simulink model "blending_tank_man"  (R2020b)
settings: Solver=FixedStepAuto  StartTime=0.0  StopTime=Inf  RelTol=1e-3
PostLoadFcn:
  | slplc.api.loadDataTypes;
undefined symbols (not defined in the file): BOOL, DINT, slplc
libraries: simulink x1, sldrtlib x1
(part 1 of 4)
CloseFcn:
  | slplc.api.clearDataTypes();
settings Model: Creator=Crystal  LastModifiedBy=Kevin

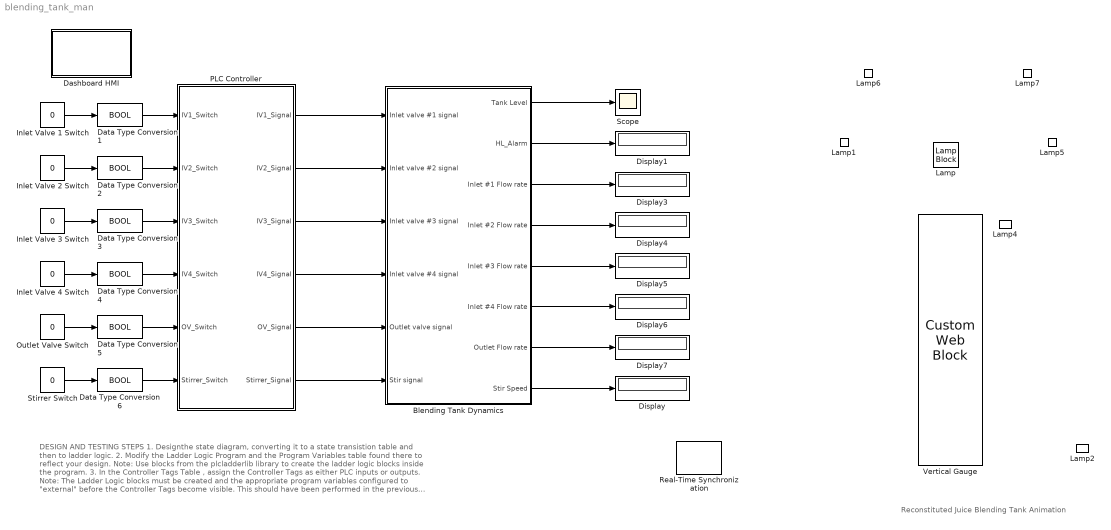
== system blending_tank_man ==
  note: Reconstituted Juice Blending Tank Animation
  note: DESIGN AND TESTING STEPS
      | 1. Designthe state diagram, converting it to a state transistion table and then to ladder logic.
      | 2. Modify the Ladder Logic Program and the Program Variables table found there to reflect your design. Note: Use blocks from the plcladderlib library to create the ladder logic blocks inside the program.
      | 3. In the Controller Tags Table , assign the Controller Tags as either PLC inputs or outputs. Note: The Ladder Logic blocks must be created and the appropriate program variables configured to "external" before the Controller Tags become visible. This should have been performed in the previous step.
      | 4. Wire the physical connections between PLC Controller outputs and the plant inputs. Note: The Controller Tags must be assigned as inputs and outputs before the I/O ports on the PLC controller block can appear. This should have been performed in the previous step.
      | 5. Wire the physical connections between the PLC controller inputs and the (a) plant (b) HMI outputs (optional).
      | 6. Optional: Design the structure of the Dashboard HMI and link the Dashboard components to the HMI outputs and the HMI inputs (from plant).
      | 7. Run the simulation . If HMI is used, control plant behaviour from Dashboard HMI .
  Blending Tank Dynamics : Subsystem
  Dashboard HMI : Subsystem
  Data Type Conversion{1..6} (6 alike) : DataTypeConversion  OutDataTypeStr=BOOL  SaturateOnIntegerOverflow=on  RndMeth=Zero
  Display{,1,3..7} (7 alike) : Display
  Inlet Valve 1 Switch : Constant  Value=0
  Inlet Valve 2 Switch : Constant  Value=0
  Inlet Valve 3 Switch : Constant  Value=0
  Inlet Valve 4 Switch : Constant  Value=0
  Lamp{,1..2,4..7} (7 alike) : LampBlock  LabelPosition=Hide
  Outlet Valve Switch : Constant  Value=0
  PLC Controller : Subsystem  TreatAsAtomicUnit=on  mask{PLCBlockType=PLCController, PLCPOUType=PLC Controller}
      mask init:
      | slplc.callbacks.initController(gcb);
      settings: OpenFcn=slplc.callbacks.openPOUBlock(gcb);
      mask Help: web([docroot '/plccoder/ref/plccontroller' '.html']);
      mask DialogControl PLCBlockTitle Prompt: PLC Controller Block
  Real-Time Synchronization : sldrtlib/Real-Time Synchronization  SampleTime=0.1  MaxMissedTicks=1000  ShowMissedTicks=off  YieldWhenWaiting=off
  Scope : Scope
  Stirrer Switch : Constant  Value=0
  Vertical Gauge : CustomWebBlock  LabelPosition=Hide  ShowInitialText=on  Configuration="{\"components\":[{\"name\":\"LinearScaleComponent\",\"settings\":{\"bounds\":{\"max\":2,\"min\":0,\"tickInterval\":0.1},\"internalTickHeightScaleFactor\":0.5,\"labelColor\":[250,245,199],\"labelFont\":{\"font\":\"Arial\",\"fontSize\":12},\"labelTransparency\":1,\"needleImage\":{\"size\":[21,75],\"src\":\"data:image\\/svg+xml;base64,PHN2ZyB4bWxucz0iaHR0cDovL3d3dy53My5vcmcvMjAwMC9zdmciIHhtbG5zOnhsaW5rPSJodHRwOi8vd3d3LnczLm9yZy8xOTk5L3hsaW5rIiB2aWV3Qm94PSIwIDAgMjEgNzUiPjxkZWZzPjxzdHlsZT4uY2xzLTF7ZmlsbDpub25lO30uY2xzLTJ7aXNvbGF0aW9uOmlzb2xhdGU7fS5jbHMtM3tjbGlwLXBhdGg6dXJsKCNjbGlwLXBhdGgpO30uY2xzLTR7b3BhY2l0eTowLjM7bWl4LWJsZW5kLW1vZGU6bXVsdGlwbHk7fS5jbHMtNXtmaWxsOiNlYjI2Mjk7fTwvc3R5bGU+PGNsaXBQYXRoIGlkPSJjbGlwLXBhdGgiIHRyYW5zZm9y ...(+1928 chars)\",\"srcOrientation\":\"horizontal\"},\"needleOffset\":[-0.01094391244870041,0],\"needleSize\":{\"height\":0.11960078534031414,\"width\":0.7589285714285714},\"position\":[0.015887605042016806,0.06986607142857143,0.8,0.9641544117647058],\"scaleColors\":[],\"scaleColorsSize\":0.2,\"showLabels\":1,\"showMinorTicks\":0,\"showSpanLine\":1,\"showTicks\":1,\"tickColor\":[250,245,200],\"tickTransparency\":1,\"valueBarColor\":[23,89,176],\"valueBarOffset\":0,\"valueBarSize\":0.23,\"valueBarTransparency\":1}},{\"name\":\"BackgroundImageComponent\",\"settings\":{\"image\":{\"size\":[101,380],\"src\":\"data:image\\/svg+xml;base64,PHN2ZyB4bWxucz0iaHR0cDovL3d3dy53My5vcmcvMjAwMC9zdmciIHZpZXdCb3g9IjAgMCAxMDEgMzgwIj48ZGVmcz48c3R5bGU+LmNscy0xe2ZpbGw6IzAwMmI0Mjt9LmNscy0ye2ZpbGw6IzQyNzA4Mjt9LmNscy0ze2ZpbGw6IzdjYTBiMjt9PC9zdHlsZT48L2RlZnM+PHRpdGxlPnZlcnRpY2FsX2dhdWdlX2JhY2tncm91bmRfMTwvdGl0bGU+PGcgaWQ9IkxheWVyXzIiIGRhdGEtbmFtZT0iTGF5ZXIgMiI+PGcgaWQ9IkxheWVyXzEtMiIgZGF0YS1uYW1lPSJMYXllciAxIj48cmVjdCBjbGFzcz0iY2xzLTEiIHg9IjExIiB5PSIxMSIgd2lkdGg9Ijc5IiBoZWlnaHQ9IjM1OCIvPjxwYXRoIGNsYXNzPSJjbHMtMiIgZD0iTTkzLDhIOFYzNzJIOTNaTTExLDM2OVYxMUg5MFYzNjlaIi8+PHBhdGggY2xhc3M9ImNscy0zIiBkPSJNMTAxLDBIMFYzODBIMTAxWk04LDM3MlY4SDkzVjM3MloiLz48L2c+PC9nPjwvc3ZnPg==\",\"srcOrientation\":\"vertical\"},\"position\":[0,0,1,1],\"scaleMode\":\"0\"}},{\"name\":\"ForegroundImageComponent\",\"settings\":{\"image\":{\"size\":[0,0],\"src\":\"default\",\"srcOrientation\":[]},\"isForeground\":1,\"position\":[0,0,1,1],\"scaleMode\":\"0\"}}],\"settings\":{\"BindingType\":\"signal\",\"aspectRatio\":0.26380368098159507,\"fixedAspectRatio\":\"on\",\"orientation\":\"vertical\"},\"type\":\"LinearGauge\"}"
  wires:
  Blending Tank Dynamics/2(HL_Alarm) -> Display1/1
  Blending Tank Dynamics/1(Tank Level) -> Scope/1
  Blending Tank Dynamics/8(Stir Speed) -> Display/1
  Blending Tank Dynamics/3(Inlet #1 Flow rate) -> Display3/1
  Blending Tank Dynamics/4(Inlet #2 Flow rate) -> Display4/1
  Blending Tank Dynamics/5(Inlet #3 Flow rate) -> Display5/1
  Blending Tank Dynamics/6(Inlet #4 Flow rate) -> Display6/1
  Blending Tank Dynamics/7(Outlet Flow rate) -> Display7/1
  PLC Controller/1(IV1_Signal) -> Blending Tank Dynamics/1(Inlet valve #1 signal)
  PLC Controller/2(IV2_Signal) -> Blending Tank Dynamics/2(Inlet valve #2 signal)
  PLC Controller/3(IV3_Signal) -> Blending Tank Dynamics/3(Inlet valve #3 signal)
  PLC Controller/4(IV4_Signal) -> Blending Tank Dynamics/4(Inlet valve #4 signal)
  PLC Controller/6(Stirrer_Signal) -> Blending Tank Dynamics/6(Stir signal)
  PLC Controller/5(OV_Signal) -> Blending Tank Dynamics/5(Outlet valve signal)
  Inlet Valve 1 Switch/1 -> Data Type Conversion1/1
  Data Type Conversion1/1 -> PLC Controller/1(IV1_Switch)
  Data Type Conversion2/1 -> PLC Controller/2(IV2_Switch)
  Inlet Valve 2 Switch/1 -> Data Type Conversion2/1
  Data Type Conversion6/1 -> PLC Controller/6(Stirrer_Switch)
  Stirrer Switch/1 -> Data Type Conversion6/1
  Outlet Valve Switch/1 -> Data Type Conversion5/1
  Data Type Conversion5/1 -> PLC Controller/5(OV_Switch)
  Inlet Valve 4 Switch/1 -> Data Type Conversion4/1
  Data Type Conversion4/1 -> PLC Controller/4(IV4_Switch)
  Inlet Valve 3 Switch/1 -> Data Type Conversion3/1
  Data Type Conversion3/1 -> PLC Controller/3(IV3_Switch)

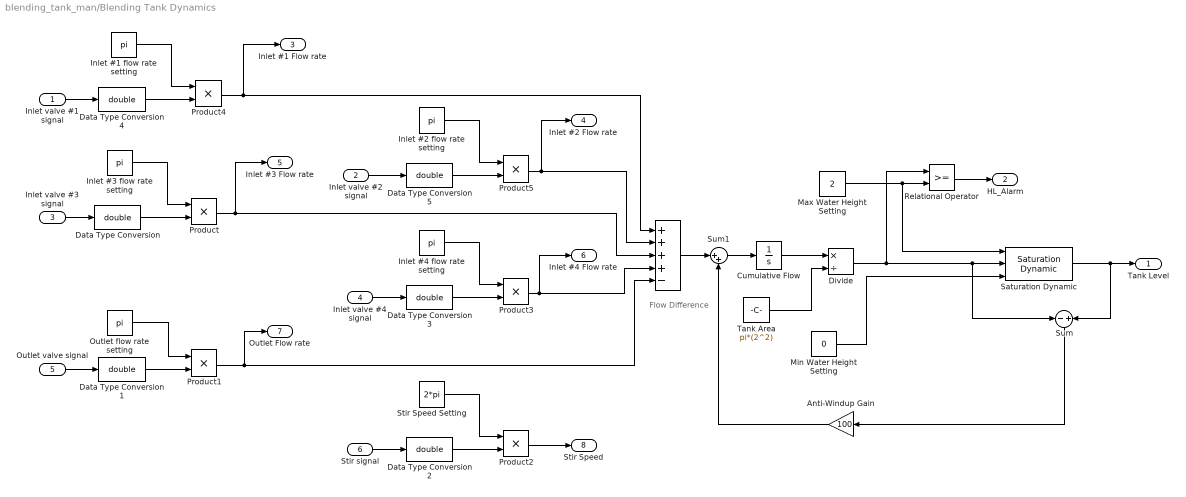
== system blending_tank_man/Blending Tank Dynamics ==
  note: Flow
      | Difference
  Inlet valve #1 signal : Inport
  Inlet valve #2 signal : Inport  Port=2
  Inlet valve #3 signal : Inport  Port=3
  Inlet valve #4 signal : Inport  Port=4
  Outlet valve signal : Inport  Port=5
  Stir signal : Inport  Port=6
  " " : Sum  Inputs=++++-  InputSameDT=on  SaturateOnIntegerOverflow=on  OutDataTypeStr=Inherit: Same as first input
  Anti-Windup Gain : Gain  Gain=100
  Cumulative Flow : Integrator
  Data Type Conversion{,1..5} (6 alike) : DataTypeConversion  OutDataTypeStr=double  SaturateOnIntegerOverflow=on  RndMeth=Zero
  Divide : Product  Inputs=*/
  Inlet #1 flow rate setting : Constant  Value=pi
  Inlet #2 flow rate setting : Constant  Value=pi
  Inlet #3 flow rate setting : Constant  Value=pi
  Inlet #4 flow rate setting : Constant  Value=pi
  Max Water Height Setting : Constant  Value=2
  "Min Water Height Setting " : Constant  Value=0
  Outlet flow rate setting : Constant  Value=pi
  Product{,1..5} (6 alike) : Product
  Relational Operator : RelationalOperator  OutDataTypeStr=boolean  RndMeth=Simplest
  Saturation Dynamic : simulink/Discontinuities/Saturation Dynamic  OutMin=[]  OutMax=[]  OutDataTypeStr=Inherit: Same as second input  OutDataType=fixdt(1, 16)  OutScaling=2^-10  DoSatur=off
  Stir Speed Setting : Constant  Value=2*pi
  Sum : Sum  Inputs=-|+
  Sum1 : Sum  Inputs=|++
  Tank Area : Constant  Value=pi*(2^2)
  Tank Level : Outport  InitialOutput=0  VectorParamsAs1DForOutWhenUnconnected=off
  HL_Alarm : Outport  Port=2
  Inlet #1 Flow rate : Outport  Port=3
  Inlet #2 Flow rate : Outport  Port=4
  Inlet #3 Flow rate : Outport  Port=5
  Inlet #4 Flow rate : Outport  Port=6
  Outlet Flow rate : Outport  Port=7
  Stir Speed : Outport  Port=8
  wires:
  Cumulative Flow/1 -> Divide/1
  Data Type Conversion/1 -> Product/2
  Inlet valve #3 signal/1 -> Data Type Conversion/1
  Outlet valve signal/1 -> Data Type Conversion1/1
  Inlet #3 flow rate setting/1 -> Product/1
  Tank Area/1 -> Divide/2
  Divide/1 -> Sum/1, Saturation Dynamic/2, Relational Operator/1
  Max Water Height Setting/1 -> Relational Operator/2, Saturation Dynamic/1
  "Min Water Height Setting "/1 -> Saturation Dynamic/3
  Relational Operator/1 -> HL_Alarm/1
  Saturation Dynamic/1 -> Sum/2, Tank Level/1
  " "/1 -> Sum1/1
  Sum1/1 -> Cumulative Flow/1
  Sum/1 -> Anti-Windup Gain/1
  Anti-Windup Gain/1 -> Sum1/2
  Stir signal/1 -> Data Type Conversion2/1
  Product2/1 -> Stir Speed/1
  Stir Speed Setting/1 -> Product2/1
  Data Type Conversion2/1 -> Product2/2
  Inlet #4 flow rate setting/1 -> Product3/1
  Inlet valve #4 signal/1 -> Data Type Conversion3/1
  Data Type Conversion3/1 -> Product3/2
  Product5/1 -> " "/2, Inlet #2 Flow rate/1
  Inlet valve #2 signal/1 -> Data Type Conversion5/1
  Inlet #2 flow rate setting/1 -> Product5/1
  Data Type Conversion5/1 -> Product5/2
  Product4/1 -> " "/1, Inlet #1 Flow rate/1
  Inlet #1 flow rate setting/1 -> Product4/1
  Inlet valve #1 signal/1 -> Data Type Conversion4/1
  Data Type Conversion4/1 -> Product4/2
  Product1/1 -> Outlet Flow rate/1, " "/5
  Product3/1 -> " "/4, Inlet #4 Flow rate/1
  Product/1 -> " "/3, Inlet #3 Flow rate/1
  Data Type Conversion1/1 -> Product1/2
  Outlet flow rate setting/1 -> Product1/1

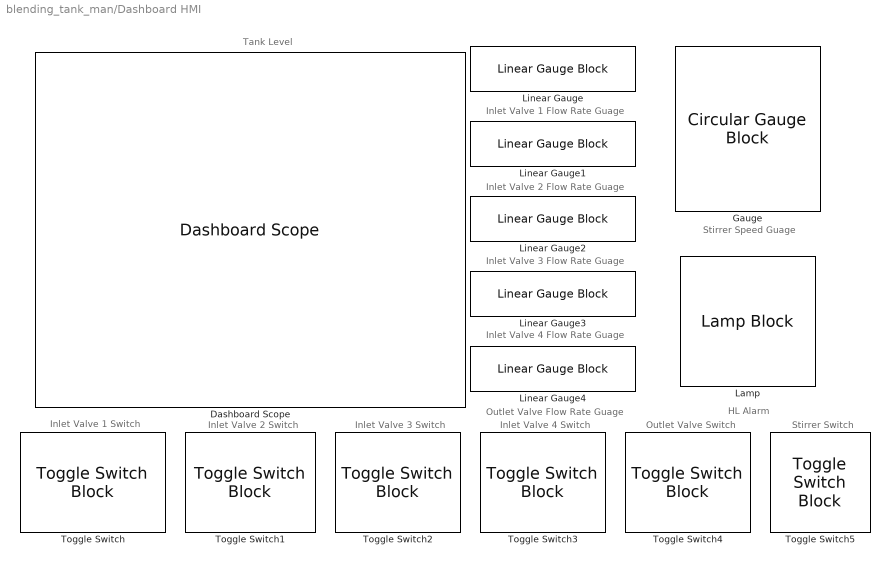
== system blending_tank_man/Dashboard HMI ==
  note: HL Alarm
  note: Stirrer Speed Guage
  note: Tank Level
  note: Inlet Valve 1 Flow Rate Guage
  note: Inlet Valve 2 Flow Rate Guage
  note: Inlet Valve 3 Flow Rate Guage
  note: Inlet Valve 4 Flow Rate Guage
  note: Outlet Valve Flow Rate Guage
  note: Inlet Valve 1 Switch
  note: Inlet Valve 2 Switch
  note: Inlet Valve 3 Switch
  note: Inlet Valve 4 Switch
  note: Outlet Valve Switch
  note: Stirrer Switch
  Dashboard Scope : DashboardScope  TimeSpan=110  Ymin=0  Ymax=2  LegendPosition=Hide  ScaleAtStop=off
  Gauge : CircularGaugeBlock  LabelPosition=Hide  ScaleMax=10  TickInterval=1
  Lamp : LampBlock  LabelPosition=Hide
  Linear Gauge{,1..4} (5 alike) : LinearGaugeBlock  LabelPosition=Hide  ScaleMax=5  TickInterval=0.5
  Toggle Switch{,1..5} (6 alike) : ToggleSwitchBlock  LabelPosition=Hide
      settings: Values={{'Off', 'On'}, [0 1]}

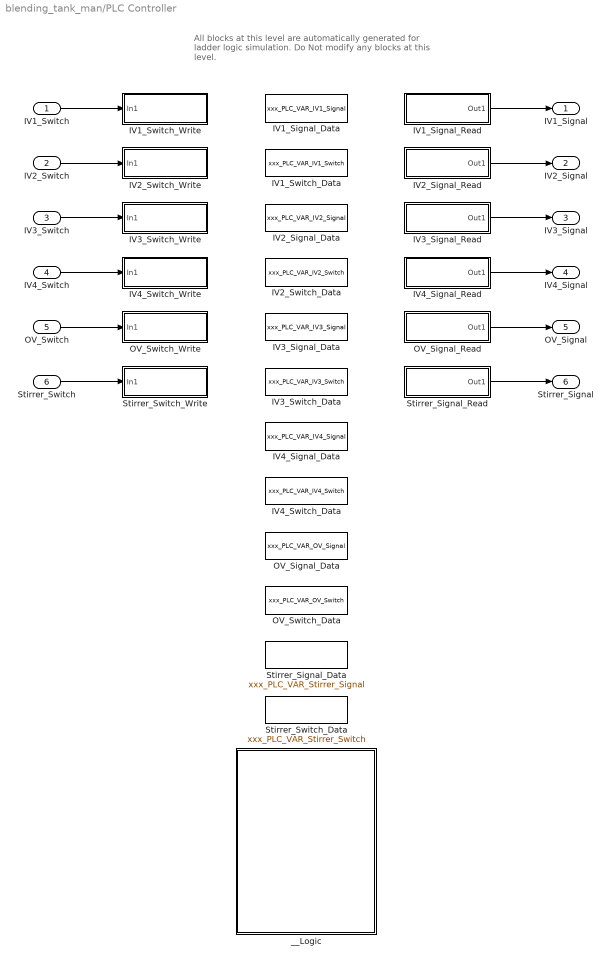
== system blending_tank_man/PLC Controller ==
  note: All blocks at this level are automatically generated for ladder logic simulation.
      | Do Not modify any blocks at this level.
  IV1_Switch : Inport  OutDataTypeStr=BOOL
  IV2_Switch : Inport  Port=2  OutDataTypeStr=BOOL
  IV3_Switch : Inport  Port=3  OutDataTypeStr=BOOL
  IV4_Switch : Inport  Port=4  OutDataTypeStr=BOOL
  OV_Switch : Inport  Port=5  OutDataTypeStr=BOOL
  Stirrer_Switch : Inport  Port=6  OutDataTypeStr=BOOL
  IV1_Signal_Data : DataStoreMemory  Tag=POUVariable  Priority=10  DataStoreName=xxx_PLC_VAR_IV1_Signal  ShowAdditionalParam=off  OutDataTypeStr=boolean  Dimensions=1
  IV1_Signal_Read : Subsystem  Priority=13  DisableCoverage=on  TreatAsAtomicUnit=on  mask{PLCOperandTag=IV1_Signal, PLCOperandExpression=xxx_PLC_VAR_IV1_Signal, PLCBlockType=VarRead, PLCPOUType=VarRead}
      mask prompts: PLCOperandTag "Operand Tag"
      mask init:
      | block = gcb;
      | maskObj = Simulink.Mask.get(block);
      | maskObj.Display = sprintf('disp(''%s'');', PLCOperandTag);
      | slplc.callbacks.initInstruction(gcb);
      mask Help: web([docroot '/plccoder/ref/varread' '.html']);
      mask DialogControl PLCBlockTitle Prompt: Variable Read
      mask Display: disp('IV1_Signal');
  IV1_Switch_Data : DataStoreMemory  Tag=POUVariable  Priority=10  DataStoreName=xxx_PLC_VAR_IV1_Switch  ShowAdditionalParam=off  OutDataTypeStr=BOOL  Dimensions=1
  IV1_Switch_Write : Subsystem  Priority=11  DisableCoverage=on  TreatAsAtomicUnit=on  mask{PLCOperandTag=IV1_Switch, PLCOperandExpression=xxx_PLC_VAR_IV1_Switch, PLCBlockType=VarWrite, PLCPOUType=VarWrite}
      mask prompts: PLCOperandTag "Operand Tag:"
      mask init:
      | slplc.callbacks.initInstruction(gcb);
      mask Help: web([docroot '/plccoder/ref/varwrite' '.html']);
      mask DialogControl PLCBlockTitle Prompt: Variable Write
      mask Display: disp(get_param(gcb, 'PLCOperandTag'));
  IV2_Signal_Data : DataStoreMemory  Tag=POUVariable  Priority=10  DataStoreName=xxx_PLC_VAR_IV2_Signal  ShowAdditionalParam=off  OutDataTypeStr=boolean  Dimensions=1
  IV2_Signal_Read : Subsystem  Priority=13  DisableCoverage=on  TreatAsAtomicUnit=on  mask{PLCOperandTag=IV2_Signal, PLCOperandExpression=xxx_PLC_VAR_IV2_Signal, PLCBlockType=VarRead, PLCPOUType=VarRead}
      mask prompts: PLCOperandTag "Operand Tag"
      mask init:
      | block = gcb;
      | maskObj = Simulink.Mask.get(block);
      | maskObj.Display = sprintf('disp(''%s'');', PLCOperandTag);
      | slplc.callbacks.initInstruction(gcb);
      mask Help: web([docroot '/plccoder/ref/varread' '.html']);
      mask DialogControl PLCBlockTitle Prompt: Variable Read
      mask Display: disp('IV2_Signal');
  IV2_Switch_Data : DataStoreMemory  Tag=POUVariable  Priority=10  DataStoreName=xxx_PLC_VAR_IV2_Switch  ShowAdditionalParam=off  OutDataTypeStr=BOOL  Dimensions=1
  IV2_Switch_Write : Subsystem  Priority=11  DisableCoverage=on  TreatAsAtomicUnit=on  mask{PLCOperandTag=IV2_Switch, PLCOperandExpression=xxx_PLC_VAR_IV2_Switch, PLCBlockType=VarWrite, PLCPOUType=VarWrite}
      mask prompts: PLCOperandTag "Operand Tag:"
      mask init:
      | slplc.callbacks.initInstruction(gcb);
      mask Help: web([docroot '/plccoder/ref/varwrite' '.html']);
      mask DialogControl PLCBlockTitle Prompt: Variable Write
      mask Display: disp(get_param(gcb, 'PLCOperandTag'));
  IV3_Signal_Data : DataStoreMemory  Tag=POUVariable  Priority=10  DataStoreName=xxx_PLC_VAR_IV3_Signal  ShowAdditionalParam=off  OutDataTypeStr=boolean  Dimensions=1
  IV3_Signal_Read : Subsystem  Priority=13  DisableCoverage=on  TreatAsAtomicUnit=on  mask{PLCOperandTag=IV3_Signal, PLCOperandExpression=xxx_PLC_VAR_IV3_Signal, PLCBlockType=VarRead, PLCPOUType=VarRead}
      mask prompts: PLCOperandTag "Operand Tag"
      mask init:
      | block = gcb;
      | maskObj = Simulink.Mask.get(block);
      | maskObj.Display = sprintf('disp(''%s'');', PLCOperandTag);
      | slplc.callbacks.initInstruction(gcb);
      mask Help: web([docroot '/plccoder/ref/varread' '.html']);
      mask DialogControl PLCBlockTitle Prompt: Variable Read
      mask Display: disp('IV3_Signal');
  IV3_Switch_Data : DataStoreMemory  Tag=POUVariable  Priority=10  DataStoreName=xxx_PLC_VAR_IV3_Switch  ShowAdditionalParam=off  OutDataTypeStr=BOOL  Dimensions=1
  IV3_Switch_Write : Subsystem  Priority=11  DisableCoverage=on  TreatAsAtomicUnit=on  mask{PLCOperandTag=IV3_Switch, PLCOperandExpression=xxx_PLC_VAR_IV3_Switch, PLCBlockType=VarWrite, PLCPOUType=VarWrite}
      mask prompts: PLCOperandTag "Operand Tag:"
      mask init:
      | slplc.callbacks.initInstruction(gcb);
      mask Help: web([docroot '/plccoder/ref/varwrite' '.html']);
      mask DialogControl PLCBlockTitle Prompt: Variable Write
      mask Display: disp(get_param(gcb, 'PLCOperandTag'));
  IV4_Signal_Data : DataStoreMemory  Tag=POUVariable  Priority=10  DataStoreName=xxx_PLC_VAR_IV4_Signal  ShowAdditionalParam=off  OutDataTypeStr=boolean  Dimensions=1
  IV4_Signal_Read : Subsystem  Priority=13  DisableCoverage=on  TreatAsAtomicUnit=on  mask{PLCOperandTag=IV4_Signal, PLCOperandExpression=xxx_PLC_VAR_IV4_Signal, PLCBlockType=VarRead, PLCPOUType=VarRead}
      mask prompts: PLCOperandTag "Operand Tag"
      mask init:
      | block = gcb;
      | maskObj = Simulink.Mask.get(block);
      | maskObj.Display = sprintf('disp(''%s'');', PLCOperandTag);
      | slplc.callbacks.initInstruction(gcb);
      mask Help: web([docroot '/plccoder/ref/varread' '.html']);
      mask DialogControl PLCBlockTitle Prompt: Variable Read
      mask Display: disp('IV4_Signal');
  IV4_Switch_Data : DataStoreMemory  Tag=POUVariable  Priority=10  DataStoreName=xxx_PLC_VAR_IV4_Switch  ShowAdditionalParam=off  OutDataTypeStr=BOOL  Dimensions=1
  IV4_Switch_Write : Subsystem  Priority=11  DisableCoverage=on  TreatAsAtomicUnit=on  mask{PLCOperandTag=IV4_Switch, PLCOperandExpression=xxx_PLC_VAR_IV4_Switch, PLCBlockType=VarWrite, PLCPOUType=VarWrite}
      mask prompts: PLCOperandTag "Operand Tag:"
      mask init:
      | slplc.callbacks.initInstruction(gcb);
      mask Help: web([docroot '/plccoder/ref/varwrite' '.html']);
      mask DialogControl PLCBlockTitle Prompt: Variable Write
      mask Display: disp(get_param(gcb, 'PLCOperandTag'));
  OV_Signal_Data : DataStoreMemory  Tag=POUVariable  Priority=10  DataStoreName=xxx_PLC_VAR_OV_Signal  ShowAdditionalParam=off  OutDataTypeStr=boolean  Dimensions=1
  OV_Signal_Read : Subsystem  Priority=13  DisableCoverage=on  TreatAsAtomicUnit=on  mask{PLCOperandTag=OV_Signal, PLCOperandExpression=xxx_PLC_VAR_OV_Signal, PLCBlockType=VarRead, PLCPOUType=VarRead}
      mask prompts: PLCOperandTag "Operand Tag"
      mask init:
      | block = gcb;
      | maskObj = Simulink.Mask.get(block);
      | maskObj.Display = sprintf('disp(''%s'');', PLCOperandTag);
      | slplc.callbacks.initInstruction(gcb);
      mask Help: web([docroot '/plccoder/ref/varread' '.html']);
      mask DialogControl PLCBlockTitle Prompt: Variable Read
      mask Display: disp('OV_Signal');
  OV_Switch_Data : DataStoreMemory  Tag=POUVariable  Priority=10  DataStoreName=xxx_PLC_VAR_OV_Switch  ShowAdditionalParam=off  OutDataTypeStr=BOOL  Dimensions=1
  OV_Switch_Write : Subsystem  Priority=11  DisableCoverage=on  TreatAsAtomicUnit=on  mask{PLCOperandTag=OV_Switch, PLCOperandExpression=xxx_PLC_VAR_OV_Switch, PLCBlockType=VarWrite, PLCPOUType=VarWrite}
      mask prompts: PLCOperandTag "Operand Tag:"
      mask init:
      | slplc.callbacks.initInstruction(gcb);
      mask Help: web([docroot '/plccoder/ref/varwrite' '.html']);
      mask DialogControl PLCBlockTitle Prompt: Variable Write
      mask Display: disp(get_param(gcb, 'PLCOperandTag'));
  Stirrer_Signal_Data : DataStoreMemory  Tag=POUVariable  Priority=10  DataStoreName=xxx_PLC_VAR_Stirrer_Signal  ShowAdditionalParam=off  OutDataTypeStr=boolean  Dimensions=1
  Stirrer_Signal_Read : Subsystem  Priority=13  DisableCoverage=on  TreatAsAtomicUnit=on  mask{PLCOperandTag=Stirrer_Signal, PLCOperandExpression=xxx_PLC_VAR_Stirrer_Signal, PLCBlockType=VarRead, PLCPOUType=VarRead}
      mask prompts: PLCOperandTag "Operand Tag"
      mask init:
      | block = gcb;
      | maskObj = Simulink.Mask.get(block);
      | maskObj.Display = sprintf('disp(''%s'');', PLCOperandTag);
      | slplc.callbacks.initInstruction(gcb);
      mask Help: web([docroot '/plccoder/ref/varread' '.html']);
      mask DialogControl PLCBlockTitle Prompt: Variable Read
      mask Display: disp('Stirrer_Signal');
  Stirrer_Switch_Data : DataStoreMemory  Tag=POUVariable  Priority=10  DataStoreName=xxx_PLC_VAR_Stirrer_Switch  ShowAdditionalParam=off  OutDataTypeStr=BOOL  Dimensions=1
  Stirrer_Switch_Write : Subsystem  Priority=11  DisableCoverage=on  TreatAsAtomicUnit=on  mask{PLCOperandTag=Stirrer_Switch, PLCOperandExpression=xxx_PLC_VAR_Stirrer_Switch, PLCBlockType=VarWrite, PLCPOUType=VarWrite}
      mask prompts: PLCOperandTag "Operand Tag:"
      mask init:
      | slplc.callbacks.initInstruction(gcb);
      mask Help: web([docroot '/plccoder/ref/varwrite' '.html']);
      mask DialogControl PLCBlockTitle Prompt: Variable Write
      mask Display: disp(get_param(gcb, 'PLCOperandTag'));
  __Logic : Subsystem  Priority=12  TreatAsAtomicUnit=on
  IV1_Signal : Outport
  IV2_Signal : Outport  Port=2
  IV3_Signal : Outport  Port=3
  IV4_Signal : Outport  Port=4
  OV_Signal : Outport  Port=5
  Stirrer_Signal : Outport  Port=6
  wires:
  IV1_Switch/1 -> IV1_Switch_Write/1(In1)
  IV2_Switch/1 -> IV2_Switch_Write/1(In1)
  IV3_Switch/1 -> IV3_Switch_Write/1(In1)
  IV4_Switch/1 -> IV4_Switch_Write/1(In1)
  OV_Switch/1 -> OV_Switch_Write/1(In1)
  Stirrer_Switch/1 -> Stirrer_Switch_Write/1(In1)
  IV1_Signal_Read/1(Out1) -> IV1_Signal/1
  IV2_Signal_Read/1(Out1) -> IV2_Signal/1
  IV3_Signal_Read/1(Out1) -> IV3_Signal/1
  IV4_Signal_Read/1(Out1) -> IV4_Signal/1
  OV_Signal_Read/1(Out1) -> OV_Signal/1
  Stirrer_Signal_Read/1(Out1) -> Stirrer_Signal/1

== system blending_tank_man/PLC Controller/IV1_Signal_Read ==
  __CoreVarRead : Subsystem  Tag=CoreVarReadBlock  DisableCoverage=on  TreatAsAtomicUnit=on  mask{PLCBlockType=CoreVarRead}
      mask init:
      | slplc.callbacks.initCoreVariable(gcb, 'read');
      mask DialogControl PLCBlockTitle Prompt: Core Variable Read
  Out1 : Outport  VectorParamsAs1DForOutWhenUnconnected=off
  wires:
  __CoreVarRead/1(y) -> Out1/1

== system blending_tank_man/PLC Controller/IV1_Switch_Write ==
  In1 : Inport
  __CoreVarWrite : Subsystem  Tag=CoreVarWriteBlock  DisableCoverage=on  TreatAsAtomicUnit=on  mask{PLCBlockType=CoreVarWrite}
      mask init:
      | slplc.callbacks.initCoreVariable(gcb, 'write');
      mask DialogControl PLCBlockTitle Prompt: Core Variable Write
  wires:
  In1/1 -> __CoreVarWrite/1(u)

== system blending_tank_man/PLC Controller/IV2_Signal_Read ==
  __CoreVarRead : Subsystem  Tag=CoreVarReadBlock  DisableCoverage=on  TreatAsAtomicUnit=on  mask{PLCBlockType=CoreVarRead}
      mask init:
      | slplc.callbacks.initCoreVariable(gcb, 'read');
      mask DialogControl PLCBlockTitle Prompt: Core Variable Read
  Out1 : Outport  VectorParamsAs1DForOutWhenUnconnected=off
  wires:
  __CoreVarRead/1(y) -> Out1/1

== system blending_tank_man/PLC Controller/IV2_Switch_Write ==
  In1 : Inport
  __CoreVarWrite : Subsystem  Tag=CoreVarWriteBlock  DisableCoverage=on  TreatAsAtomicUnit=on  mask{PLCBlockType=CoreVarWrite}
      mask init:
      | slplc.callbacks.initCoreVariable(gcb, 'write');
      mask DialogControl PLCBlockTitle Prompt: Core Variable Write
  wires:
  In1/1 -> __CoreVarWrite/1(u)

== system blending_tank_man/PLC Controller/IV3_Signal_Read ==
  __CoreVarRead : Subsystem  Tag=CoreVarReadBlock  DisableCoverage=on  TreatAsAtomicUnit=on  mask{PLCBlockType=CoreVarRead}
      mask init:
      | slplc.callbacks.initCoreVariable(gcb, 'read');
      mask DialogControl PLCBlockTitle Prompt: Core Variable Read
  Out1 : Outport  VectorParamsAs1DForOutWhenUnconnected=off
  wires:
  __CoreVarRead/1(y) -> Out1/1

== system blending_tank_man/PLC Controller/IV3_Switch_Write ==
  In1 : Inport
  __CoreVarWrite : Subsystem  Tag=CoreVarWriteBlock  DisableCoverage=on  TreatAsAtomicUnit=on  mask{PLCBlockType=CoreVarWrite}
      mask init:
      | slplc.callbacks.initCoreVariable(gcb, 'write');
      mask DialogControl PLCBlockTitle Prompt: Core Variable Write
  wires:
  In1/1 -> __CoreVarWrite/1(u)

== system blending_tank_man/PLC Controller/IV4_Signal_Read ==
  __CoreVarRead : Subsystem  Tag=CoreVarReadBlock  DisableCoverage=on  TreatAsAtomicUnit=on  mask{PLCBlockType=CoreVarRead}
      mask init:
      | slplc.callbacks.initCoreVariable(gcb, 'read');
      mask DialogControl PLCBlockTitle Prompt: Core Variable Read
  Out1 : Outport  VectorParamsAs1DForOutWhenUnconnected=off
  wires:
  __CoreVarRead/1(y) -> Out1/1

== system blending_tank_man/PLC Controller/IV4_Switch_Write ==
  In1 : Inport
  __CoreVarWrite : Subsystem  Tag=CoreVarWriteBlock  DisableCoverage=on  TreatAsAtomicUnit=on  mask{PLCBlockType=CoreVarWrite}
      mask init:
      | slplc.callbacks.initCoreVariable(gcb, 'write');
      mask DialogControl PLCBlockTitle Prompt: Core Variable Write
  wires:
  In1/1 -> __CoreVarWrite/1(u)

== system blending_tank_man/PLC Controller/OV_Signal_Read ==
  __CoreVarRead : Subsystem  Tag=CoreVarReadBlock  DisableCoverage=on  TreatAsAtomicUnit=on  mask{PLCBlockType=CoreVarRead}
      mask init:
      | slplc.callbacks.initCoreVariable(gcb, 'read');
      mask DialogControl PLCBlockTitle Prompt: Core Variable Read
  Out1 : Outport  VectorParamsAs1DForOutWhenUnconnected=off
  wires:
  __CoreVarRead/1(y) -> Out1/1

== system blending_tank_man/PLC Controller/OV_Switch_Write ==
  In1 : Inport
  __CoreVarWrite : Subsystem  Tag=CoreVarWriteBlock  DisableCoverage=on  TreatAsAtomicUnit=on  mask{PLCBlockType=CoreVarWrite}
      mask init:
      | slplc.callbacks.initCoreVariable(gcb, 'write');
      mask DialogControl PLCBlockTitle Prompt: Core Variable Write
  wires:
  In1/1 -> __CoreVarWrite/1(u)

== system blending_tank_man/PLC Controller/Stirrer_Signal_Read ==
  __CoreVarRead : Subsystem  Tag=CoreVarReadBlock  DisableCoverage=on  TreatAsAtomicUnit=on  mask{PLCBlockType=CoreVarRead}
      mask init:
      | slplc.callbacks.initCoreVariable(gcb, 'read');
      mask DialogControl PLCBlockTitle Prompt: Core Variable Read
  Out1 : Outport  VectorParamsAs1DForOutWhenUnconnected=off
  wires:
  __CoreVarRead/1(y) -> Out1/1

== system blending_tank_man/PLC Controller/Stirrer_Switch_Write ==
  In1 : Inport
  __CoreVarWrite : Subsystem  Tag=CoreVarWriteBlock  DisableCoverage=on  TreatAsAtomicUnit=on  mask{PLCBlockType=CoreVarWrite}
      mask init:
      | slplc.callbacks.initCoreVariable(gcb, 'write');
      mask DialogControl PLCBlockTitle Prompt: Core Variable Write
  wires:
  In1/1 -> __CoreVarWrite/1(u)

== system blending_tank_man/PLC Controller/__Logic ==
  Controller Tags : Subsystem  Tag=ControllerVariableSS  DisableCoverage=on  TreatAsAtomicUnit=on  mask{PLCVarIV1_SwitchName=IV1_Switch, PLCVarIV1_SwitchAddress=<empty>, PLCVarIV1_SwitchMapping=Input Symbol, PLCVarIV1_SwitchPortIndex=1, PLCVarIV1_SwitchDataType=BOOL, PLCVarIV1_SwitchSize=1, PLCVarIV1_SwitchInitialValue=0, PLCVarIV1_SwitchToDelete=off, PLCVarIV2_SwitchName=IV2_Switch, PLCVarIV2_SwitchAddress=<empty>, PLCVarIV2_SwitchMapping=Input Symbol, PLCVarIV2_SwitchPortIndex=2, PLCVarIV2_SwitchDataType=BOOL, PLCVarIV2_SwitchSize=1, PLCVarIV2_SwitchInitialValue=0, PLCVarIV2_SwitchToDelete=off, PLCVarIV3_SwitchName=IV3_Switch, PLCVarIV3_SwitchAddress=<empty>, PLCVarIV3_SwitchMapping=Input Symbol, PLCVarIV3_SwitchPortIndex=3, PLCVarIV3_SwitchDataType=BOOL, PLCVarIV3_SwitchSize=1, PLCVarIV3_SwitchInitialValue=0, PLCVarIV3_SwitchToDelete=off, PLCVarIV4_SwitchName=IV4_Switch, PLCVarIV4_SwitchAddress=<empty>, PLCVarIV4_SwitchMapping=Input Symbol, PLCVarIV4_SwitchPortIndex=4, PLCVarIV4_SwitchDataType=BOOL, PLCVarIV4_SwitchSize=1, PLCVarIV4_SwitchInitialValue=0, PLCVarIV4_SwitchToDelete=off, PLCVarOV_SwitchName=OV_Switch, PLCVarOV_SwitchAddress=<empty>, PLCVarOV_SwitchMapping=Input Symbol, PLCVarOV_SwitchPortIndex=5, PLCVarOV_SwitchDataType=BOOL, PLCVarOV_SwitchSize=1, PLCVarOV_SwitchInitialValue=0, PLCVarOV_SwitchToDelete=off, PLCVarStirrer_SwitchName=Stirrer_Switch, PLCVarStirrer_SwitchAddress=<empty>, PLCVarStirrer_SwitchMapping=Input Symbol, PLCVarStirrer_SwitchPortIndex=6, PLCVarStirrer_SwitchDataType=BOOL, PLCVarStirrer_SwitchSize=1, PLCVarStirrer_SwitchInitialValue=0, PLCVarStirrer_SwitchToDelete=off, PLCVarIV1_SignalName=IV1_Signal, PLCVarIV1_SignalAddress=<empty>, PLCVarIV1_SignalMapping=Output Symbol, PLCVarIV1_SignalPortIndex=1, PLCVarIV1_SignalDataType=boolean, PLCVarIV1_SignalSize=1, PLCVarIV1_SignalInitialValue=0, PLCVarIV1_SignalToDelete=off, PLCVarIV2_SignalName=IV2_Signal, PLCVarIV2_SignalAddress=<empty>, PLCVarIV2_SignalMapping=Output Symbol, PLCVarIV2_SignalPortIndex=2, PLCVarIV2_SignalDataType=boolean, PLCVarIV2_SignalSize=1, PLCVarIV2_SignalInitialValue=0, PLCVarIV2_SignalToDelete=off, PLCVarIV3_SignalName=IV3_Signal, PLCVarIV3_SignalAddress=<empty>, PLCVarIV3_SignalMapping=Output Symbol, PLCVarIV3_SignalPortIndex=3, PLCVarIV3_SignalDataType=boolean, PLCVarIV3_SignalSize=1, PLCVarIV3_SignalInitialValue=0, PLCVarIV3_SignalToDelete=off, PLCVarIV4_SignalName=IV4_Signal, PLCVarIV4_SignalAddress=<empty>, PLCVarIV4_SignalMapping=Output Symbol, PLCVarIV4_SignalPortIndex=4, PLCVarIV4_SignalDataType=boolean, PLCVarIV4_SignalSize=1, PLCVarIV4_SignalInitialValue=0, PLCVarIV4_SignalToDelete=off, PLCVarOV_SignalName=OV_Signal, PLCVarOV_SignalAddress=<empty>, PLCVarOV_SignalMapping=Output Symbol, PLCVarOV_SignalPortIndex=5, PLCVarOV_SignalDataType=boolean, PLCVarOV_SignalSize=1, PLCVarOV_SignalInitialValue=0, PLCVarOV_SignalToDelete=off, PLCVarStirrer_SignalName=Stirrer_Signal, PLCVarStirrer_SignalAddress=<empty>, PLCVarStirrer_SignalMapping=Output Symbol, PLCVarStirrer_SignalPortIndex=6, PLCVarStirrer_SignalDataType=boolean, PLCVarStirrer_SignalSize=1, PLCVarStirrer_SignalInitialValue=0, PLCVarStirrer_SignalToDelete=off}
      mask init:
      | slplc.callbacks.initControllerVarSS(gcb);
      settings: OpenFcn=slplc.callbacks.openControllerVariableSS(gcb);
      mask Help: web([docroot '/plccoder/ref/controllertags' '.html']);
      mask TypeOptions PLCVarIV1_SwitchMapping: Global Variable | Input Symbol | Output Symbol
      mask Callback PLCVarIV1_SwitchMapping: slplc.callbacks.updateControllerVarSS(gcb);
      mask TypeOptions PLCVarIV1_SwitchPortIndex: 1 | 2 | 3 | 4 | 5 | 6 | 7 | 8 | 9 | 10 | 11 | 12
      mask TypeOptions PLCVarIV2_SwitchMapping: Global Variable | Input Symbol | Output Symbol
      mask Callback PLCVarIV2_SwitchMapping: slplc.callbacks.updateControllerVarSS(gcb);
      mask TypeOptions PLCVarIV2_SwitchPortIndex: 1 | 2 | 3 | 4 | 5 | 6 | 7 | 8 | 9 | 10 | 11 | 12
      mask TypeOptions PLCVarIV3_SwitchMapping: Global Variable | Input Symbol | Output Symbol
      mask Callback PLCVarIV3_SwitchMapping: slplc.callbacks.updateControllerVarSS(gcb);
      mask TypeOptions PLCVarIV3_SwitchPortIndex: 1 | 2 | 3 | 4 | 5 | 6 | 7 | 8 | 9 | 10 | 11 | 12
      mask TypeOptions PLCVarIV4_SwitchMapping: Global Variable | Input Symbol | Output Symbol
      mask Callback PLCVarIV4_SwitchMapping: slplc.callbacks.updateControllerVarSS(gcb);
      mask TypeOptions PLCVarIV4_SwitchPortIndex: 1 | 2 | 3 | 4 | 5 | 6 | 7 | 8 | 9 | 10 | 11 | 12
      mask TypeOptions PLCVarOV_SwitchMapping: Global Variable | Input Symbol | Output Symbol
      mask Callback PLCVarOV_SwitchMapping: slplc.callbacks.updateControllerVarSS(gcb);
      mask TypeOptions PLCVarOV_SwitchPortIndex: 1 | 2 | 3 | 4 | 5 | 6 | 7 | 8 | 9 | 10 | 11 | 12
      mask TypeOptions PLCVarStirrer_SwitchMapping: Global Variable | Input Symbol | Output Symbol
      mask Callback PLCVarStirrer_SwitchMapping: slplc.callbacks.updateControllerVarSS(gcb);
      mask TypeOptions PLCVarStirrer_SwitchPortIndex: 1 | 2 | 3 | 4 | 5 | 6 | 7 | 8 | 9 | 10 | 11 | 12
      mask TypeOptions PLCVarIV1_SignalMapping: Global Variable | Input Symbol | Output Symbol
      mask Callback PLCVarIV1_SignalMapping: slplc.callbacks.updateControllerVarSS(gcb);
      mask TypeOptions PLCVarIV1_SignalPortIndex: 1 | 2 | 3 | 4 | 5 | 6 | 7 | 8 | 9 | 10 | 11 | 12
      mask TypeOptions PLCVarIV2_SignalMapping: Global Variable | Input Symbol | Output Symbol
      mask Callback PLCVarIV2_SignalMapping: slplc.callbacks.updateControllerVarSS(gcb);
      mask TypeOptions PLCVarIV2_SignalPortIndex: 1 | 2 | 3 | 4 | 5 | 6 | 7 | 8 | 9 | 10 | 11 | 12
      mask TypeOptions PLCVarIV3_SignalMapping: Global Variable | Input Symbol | Output Symbol
      mask Callback PLCVarIV3_SignalMapping: slplc.callbacks.updateControllerVarSS(gcb);
      mask TypeOptions PLCVarIV3_SignalPortIndex: 1 | 2 | 3 | 4 | 5 | 6 | 7 | 8 | 9 | 10 | 11 | 12
      mask TypeOptions PLCVarIV4_SignalMapping: Global Variable | Input Symbol | Output Symbol
      mask Callback PLCVarIV4_SignalMapping: slplc.callbacks.updateControllerVarSS(gcb);
      mask TypeOptions PLCVarIV4_SignalPortIndex: 1 | 2 | 3 | 4 | 5 | 6 | 7 | 8 | 9 | 10 | 11 | 12
      mask TypeOptions PLCVarOV_SignalMapping: Global Variable | Input Symbol | Output Symbol
      mask Callback PLCVarOV_SignalMapping: slplc.callbacks.updateControllerVarSS(gcb);
      mask TypeOptions PLCVarOV_SignalPortIndex: 1 | 2 | 3 | 4 | 5 | 6 | 7 | 8 | 9 | 10 | 11 | 12
      mask TypeOptions PLCVarStirrer_SignalMapping: Global Variable | Input Symbol | Output Symbol
      mask Callback PLCVarStirrer_SignalMapping: slplc.callbacks.updateControllerVarSS(gcb);
      mask TypeOptions PLCVarStirrer_SignalPortIndex: 1 | 2 | 3 | 4 | 5 | 6 | 7 | 8 | 9 | 10 | 11 | 12
      mask DialogControl PLCBlockTitle Prompt: Global Variable and Symbol Spreadsheet
      mask DialogControl PLCVarListHeaderName Prompt: Name
      mask DialogControl PLCVarListHeaderAddress Prompt: Address (At)
      mask DialogControl PLCVarListHeaderMapping Prompt: Mapping Type
      mask DialogControl PLCVarListHeaderPortIndex Prompt: Port
      mask DialogControl PLCVarListHeaderDataType Prompt: Data Type
      mask DialogControl PLCVarListHeaderSize Prompt: Size
      mask DialogControl PLCVarListHeaderInitialValue Prompt: Initial Value
      mask DialogControl PLCVarListHeaderToDelete Prompt: Delete
  Task : Subsystem  TreatAsAtomicUnit=on  mask{PLCBlockType=Task, PLCPOUType=Task, PLCTaskWatchDog=0}
      mask init:
      | slplc.callbacks.initTask(gcb);
      settings: OpenFcn=slplc.callbacks.openTaskBlock(gcb);
      mask Help: web([docroot '/plccoder/ref/task' '.html']);
      mask DialogControl PLCBlockTitle Prompt: Task
  Up to Parent POU : Subsystem  DisableCoverage=on  TreatAsAtomicUnit=on  mask{PLCBlockType=OpenParentPOU}
      settings: OpenFcn=slplc.callbacks.openParentPOUBlock(gcb);
      mask Help: web([docroot '/plccoder/ref/uptoparentpou' '.html']);
      mask DialogControl PLCBlockTitle Prompt: Add Single Rung

== system blending_tank_man/PLC Controller/IV1_Signal_Read/__CoreVarRead ==
  DataRead : DataStoreRead  DataStoreName=xxx_PLC_VAR_IV1_Signal
  y : Outport  VectorParamsAs1DForOutWhenUnconnected=off
  wires:
  DataRead/1 -> y/1

== system blending_tank_man/PLC Controller/IV1_Switch_Write/__CoreVarWrite ==
  u : Inport
  DataWrite : DataStoreWrite  DataStoreName=xxx_PLC_VAR_IV1_Switch
  wires:
  u/1 -> DataWrite/1

== system blending_tank_man/PLC Controller/IV2_Signal_Read/__CoreVarRead ==
  DataRead : DataStoreRead  DataStoreName=xxx_PLC_VAR_IV2_Signal
  y : Outport  VectorParamsAs1DForOutWhenUnconnected=off
  wires:
  DataRead/1 -> y/1

== system blending_tank_man/PLC Controller/IV2_Switch_Write/__CoreVarWrite ==
  u : Inport
  DataWrite : DataStoreWrite  DataStoreName=xxx_PLC_VAR_IV2_Switch
  wires:
  u/1 -> DataWrite/1

== system blending_tank_man/PLC Controller/IV3_Signal_Read/__CoreVarRead ==
  DataRead : DataStoreRead  DataStoreName=xxx_PLC_VAR_IV3_Signal
  y : Outport  VectorParamsAs1DForOutWhenUnconnected=off
  wires:
  DataRead/1 -> y/1

== system blending_tank_man/PLC Controller/IV3_Switch_Write/__CoreVarWrite ==
  u : Inport
  DataWrite : DataStoreWrite  DataStoreName=xxx_PLC_VAR_IV3_Switch
  wires:
  u/1 -> DataWrite/1

== system blending_tank_man/PLC Controller/IV4_Signal_Read/__CoreVarRead ==
  DataRead : DataStoreRead  DataStoreName=xxx_PLC_VAR_IV4_Signal
  y : Outport  VectorParamsAs1DForOutWhenUnconnected=off
  wires:
  DataRead/1 -> y/1

== system blending_tank_man/PLC Controller/IV4_Switch_Write/__CoreVarWrite ==
  u : Inport
  DataWrite : DataStoreWrite  DataStoreName=xxx_PLC_VAR_IV4_Switch
  wires:
  u/1 -> DataWrite/1

== system blending_tank_man/PLC Controller/OV_Signal_Read/__CoreVarRead ==
  DataRead : DataStoreRead  DataStoreName=xxx_PLC_VAR_OV_Signal
  y : Outport  VectorParamsAs1DForOutWhenUnconnected=off
  wires:
  DataRead/1 -> y/1

== system blending_tank_man/PLC Controller/OV_Switch_Write/__CoreVarWrite ==
  u : Inport
  DataWrite : DataStoreWrite  DataStoreName=xxx_PLC_VAR_OV_Switch
  wires:
  u/1 -> DataWrite/1

== system blending_tank_man/PLC Controller/Stirrer_Signal_Read/__CoreVarRead ==
  DataRead : DataStoreRead  DataStoreName=xxx_PLC_VAR_Stirrer_Signal
  y : Outport  VectorParamsAs1DForOutWhenUnconnected=off
  wires:
  DataRead/1 -> y/1

== system blending_tank_man/PLC Controller/Stirrer_Switch_Write/__CoreVarWrite ==
  u : Inport
  DataWrite : DataStoreWrite  DataStoreName=xxx_PLC_VAR_Stirrer_Switch
  wires:
  u/1 -> DataWrite/1

== system blending_tank_man/PLC Controller/__Logic/Controller Tags ==

== system blending_tank_man/PLC Controller/__Logic/Task ==
  Program : Subsystem  TreatAsAtomicUnit=on  mask{PLCPOUType=Program, PLCPOULanguage=LD, PLCBlockType=LDProgram}
      mask prompts: PLCPOUType "POU Type:"
      mask init:
      | slplc.callbacks.initProgram(gcb);
      settings: OpenFcn=slplc.callbacks.openPOUBlock(gcb);
      mask Help: web([docroot '/plccoder/ref/program' '.html']);
      mask DialogControl PLCBlockTitle Prompt: Program
      mask DialogControl PLCEditPOU Prompt: Edit POU
      mask DialogControl PLCEditInterface Prompt: Edit Variables
  Up to Parent POU : Subsystem  DisableCoverage=on  TreatAsAtomicUnit=on  mask{PLCBlockType=OpenParentPOU}
      settings: OpenFcn=slplc.callbacks.openParentPOUBlock(gcb);
      mask Help: web([docroot '/plccoder/ref/uptoparentpou' '.html']);
      mask DialogControl PLCBlockTitle Prompt: Add Single Rung

== system blending_tank_man/PLC Controller/__Logic/Up to Parent POU ==

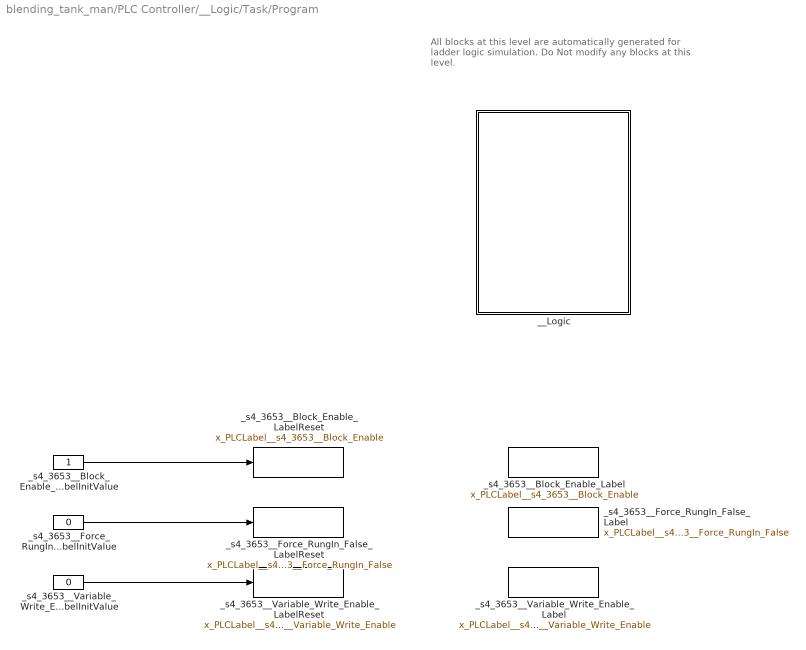
== system blending_tank_man/PLC Controller/__Logic/Task/Program ==
  note: All blocks at this level are automatically generated for ladder logic simulation.
      | Do Not modify any blocks at this level.
  __Logic : Subsystem  Priority=12  TreatAsAtomicUnit=on
  _s4_3653__Block_Enable_Label : DataStoreMemory  Priority=10  DataStoreName=x_PLCLabel__s4_3653__Block_Enable  InitialValue=1  ShowAdditionalParam=off  OutDataTypeStr=BOOL  Dimensions=1
  _s4_3653__Block_Enable_LabelInitValue : Constant  OutDataTypeStr=BOOL
  _s4_3653__Block_Enable_LabelReset : DataStoreWrite  Priority=11  DataStoreName=x_PLCLabel__s4_3653__Block_Enable
  _s4_3653__Force_RungIn_False_Label : DataStoreMemory  Priority=10  DataStoreName=x_PLCLabel__s4_3653__Force_RungIn_False  ShowAdditionalParam=off  OutDataTypeStr=BOOL  Dimensions=1
  _s4_3653__Force_RungIn_False_LabelInitValue : Constant  Value=0  OutDataTypeStr=BOOL
  _s4_3653__Force_RungIn_False_LabelReset : DataStoreWrite  Priority=11  DataStoreName=x_PLCLabel__s4_3653__Force_RungIn_False
  _s4_3653__Variable_Write_Enable_Label : DataStoreMemory  Priority=10  DataStoreName=x_PLCLabel__s4_3653__Variable_Write_Enable  ShowAdditionalParam=off  OutDataTypeStr=BOOL  Dimensions=1
  _s4_3653__Variable_Write_Enable_LabelInitValue : Constant  Value=0  OutDataTypeStr=BOOL
  _s4_3653__Variable_Write_Enable_LabelReset : DataStoreWrite  Priority=11  DataStoreName=x_PLCLabel__s4_3653__Variable_Write_Enable
  wires:
  _s4_3653__Block_Enable_LabelInitValue/1 -> _s4_3653__Block_Enable_LabelReset/1
  _s4_3653__Variable_Write_Enable_LabelInitValue/1 -> _s4_3653__Variable_Write_Enable_LabelReset/1
  _s4_3653__Force_RungIn_False_LabelInitValue/1 -> _s4_3653__Force_RungIn_False_LabelReset/1

== system blending_tank_man/PLC Controller/__Logic/Task/Up to Parent POU ==
